simulink model "Tricopter_Controlled_development"  (R2015a)
settings: Solver=ode2  SolverMode=SingleTasking  StartTime=0.0  StopTime=inf  FixedStep=T_sim  RelTol=1e-3
values from neighbouring files (symbols this model uses):
  A_l_max_x = sqrt( (A_z_max)^2  -  g^2  )    [Run3Copter.m]
  A_l_max_y = g*tand(15)    [Run3Copter.m]
  A_x = 0.015    [SetupComplete.m]
  A_y = A_x    (= 0.015)    [SetupComplete.m]
  A_z = 0.16    [SetupComplete.m]
  A_z_max = Max_Thrust*3/m    [Run3Copter.m]
  Alt_0 = input(' Give the initial altitude (m): ')    [Run3Copter.m]
  C_x = 1.2    [SetupComplete.m]
  C_y = C_x    (= 1.2)    [SetupComplete.m]
  C_z = 2.2    [SetupComplete.m]
  CG_0 = [0,0,0.02]'    [SetupComplete.m]
  epsilon = 0.01    [Run3Copter.m]
  eta_23 = deg2rad(-1.3)    [Run3Copter.m]
  g = 9.81    [SetupComplete.m]
  h = 0.08    [SetupComplete.m]
  h_M = 0.064    [SetupComplete.m]
  I_BAC_0 = [ Ix,0,Ixz;0,Iy,0;Ixz,0,Iz]    [SetupComplete.m]
  Initial_Omegas = Omega_hover    [Run3Copter.m]
  Initial_Torques = Torque_hover    [Run3Copter.m]
  Ix = 0.103    [SetupComplete.m]
  Iy = 0.147    [SetupComplete.m]
  Iz = 0.237    [SetupComplete.m]
  l = 0.345    [SetupComplete.m]
  l_arm = 0.264    [SetupComplete.m]
  latitude = 52.071118    [Run3Copter.m]
  longitude = -0.627404    [Run3Copter.m]
  m = 3.51    [SetupComplete.m]
  m_0 = 2.61    [SetupComplete.m]
  m_M = 0.300    (= 0.3)    [SetupComplete.m]
  rho = 1.15    [SetupComplete.m]
  Rotation_sign = [ 1,-1,-1]    [SetupComplete.m]
  T_ctrl = 0.02    [Run3Copter.m]
  T_sim = 0.01    [Run3Copter.m]
  throtle_1 = 0*0.745    (= 0)    [Run3Copter.m]
  throtle_23 = throtle_1/cos(eta_23)    [Run3Copter.m]
  v_i0 = sqrt( 1/3*m*g/(2*rho*pi*R^2)  )    [SetupComplete.m]
undefined symbols (not defined in the file or in its folder): DOWN_0, EAST_0, Newton, NORTH_0, P_0, Q_0, R_0, Raphson, U_0, V_0, W_0
libraries: Adaptive_FaultTolerantControl x30, XXCopter_Control x23, simulink_extras x17, XXCopter x5, simulink x2, qcatlib x1, XXCopter_C x1
(part 2 of 4)

== system Tricopter_Controlled_development/TriCopter FCS development/Build Servos PWM ==
  note: Control input
      | Rango
      | Direccion rot/Dir servos
      | Rango del servo
      |
      | eta_1 (rad) (Pan arm 1)
      | -165,165
      | -1
      | 330: -165,165
      |
      | gamma_1 (rad) (Tilt arm 1)
      | -90,15
      | -1
      | 180:-90,90 ó 330: -165,165
      |
      | eta_2 (rad) (Pan arm 2)
      | -165,165
      | -1
      | 330: -165,165
      |
      | gamma_2 (rad) (Tilt arm 2)
      | -15,90
      | 1
      | 180:-90,90
      |
      | eta_3 (rad) (Pan arm 3)
      | -165,165
      | 1
      | 330:-165,165
      |
      | gamma_3 (rad) (Tilt arm 3)
      | -90,15
      | -1
      | 180:-90,90
  signals servos in : Inport
  Demux : Demux  Outputs=6
  Mux : Mux  Inputs=6
  Signal2PWM1 : XXCopter_Control/Signal2PWM  b=deg2rad(165)  d=-deg2rad(165)  a=2100  c=900
  Signal2PWM2 : XXCopter_Control/Signal2PWM  b=deg2rad(90)  d=-deg2rad(90)  a=2100  c=900
  Signal2PWM3 : XXCopter_Control/Signal2PWM  b=deg2rad(90)  d=-deg2rad(90)  a=2100  c=900
  Signal2PWM4 : XXCopter_Control/Signal2PWM  b=deg2rad(90)  d=-deg2rad(90)  a=2100  c=900
  Signal2PWM5 : XXCopter_Control/Signal2PWM  b=deg2rad(165)  d=-deg2rad(165)  a=2100  c=900
  Signal2PWM6 : XXCopter_Control/Signal2PWM  b=deg2rad(165)  d=-deg2rad(165)  a=2100  c=900
  Unary Minus{,1..3} (4 alike) : UnaryMinus
  PWM_us servos out : Outport
  wires:
  signals servos in/1 -> Demux/1
  Demux/1 -> Unary Minus/1
  Demux/2 -> Unary Minus1/1
  Demux/3 -> Unary Minus2/1
  Demux/6 -> Unary Minus3/1
  Unary Minus3/1 -> Signal2PWM3/1
  Demux/5 -> Signal2PWM6/1
  Demux/4 -> Signal2PWM4/1
  Unary Minus2/1 -> Signal2PWM5/1
  Unary Minus1/1 -> Signal2PWM2/1
  Unary Minus/1 -> Signal2PWM1/1
  Signal2PWM1/1 -> Mux/1
  Signal2PWM2/1 -> Mux/2
  Signal2PWM5/1 -> Mux/3
  Signal2PWM4/1 -> Mux/4
  Signal2PWM6/1 -> Mux/5
  Signal2PWM3/1 -> Mux/6
  Mux/1 -> PWM_us servos out/1

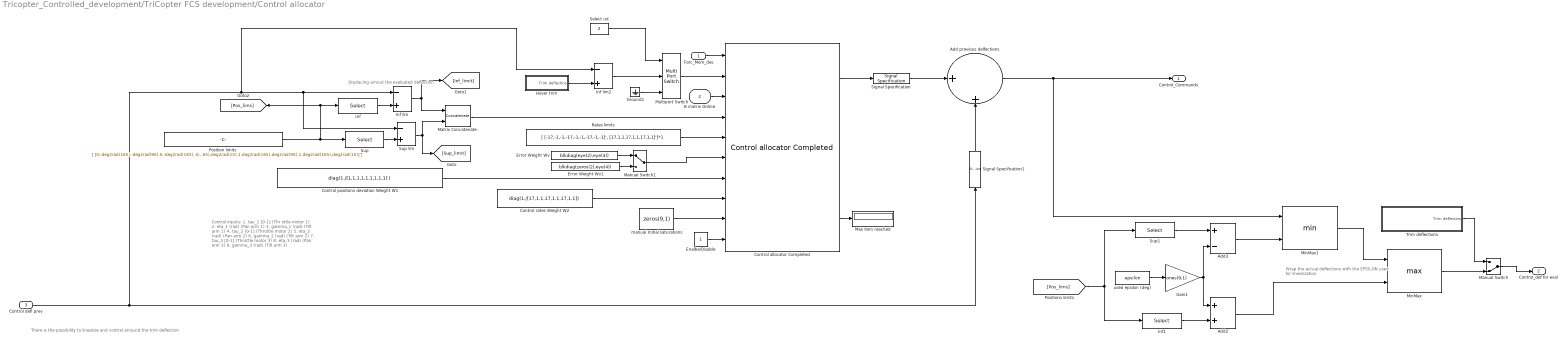
== system Tricopter_Controlled_development/TriCopter FCS development/Control allocator ==
  note: There is the possibility to linearize and control arround the trim deflection
  note: Wrap the actual deflections with the EPSILON
      |  used for linearization
  note: Displacing arroud the evaluated deflection
  note: Control inputs:
      | 1. tau_1 [0-1] (Thr ottle motor 1)
      | 2. eta_1 (rad)  (Pan arm 1)
      | 3. gamma_1 (rad)  (Tilt arm 1)
      |
      | 4. tau_2 [0-1] (Throttle motor 2)
      | 5. eta_2 (rad)  (Pan arm 2)
      | 6. gamma_2 (rad)  (Tilt arm 2)
      |
      | 7. tau_3 [0-1] (Throttle motor 3)
      | 8. eta_3 (rad)  (Pan arm  3)
      | 9. gamma_3 (rad)  (Tilt arm 3)
  Forc_Mom_des : Inport
  B matrix Online : Inport  Port=2
  Control defl prev : Inport  Port=3
  Add previous delfections : Sum  Inputs=|++
  Add2 : Sum
  Add3 : Sum  Inputs=+-
  "Control allocator Completed " : qcatlib/Control allocator Completed   alg=WLS  CA_type=QP  iter_max=100  gamma=1  k_B=6  m_B=9  T=T_ctrl  tol=1e-5
  Control positions deviation Weight W1 : Constant  Value=diag(1./[1,1,1,1,1,1,1,1,1] )
  Control rates Weight W2 : Constant  Value=diag(1./[17,1,1,17,1,1,17,1,1])
  Enalbe/Disable : Constant
  Error Weight Wv : Constant  Value=blkdiag(eye(2),eye(4))
  Error Weight Wv1 : Constant  Value=blkdiag(zeros(2),eye(4))
  Gain1 : Gain  Gain=ones(9,1)
  Ground1 : Ground
  Hover trim : Subsystem  TreatAsAtomicUnit=on
  Inf : Selector  NumberOfDimensions=2  InputPortWidth=3  IndexOptions=Index vector (dialog),Index vector (dialog)  Indices=[1:9],1  OutputSizes=1,1
  Inf lim : Sum  Inputs=-+
  Inf lim2 : Sum  Inputs=-+
  Inf1 : Selector  NumberOfDimensions=2  InputPortWidth=3  IndexOptions=Index vector (dialog),Index vector (dialog)  Indices=[1:9],1  OutputSizes=1,1
  Manual Switch : ManualSwitch  CurrentSetting=0
  Manual Switch1 : ManualSwitch
  Matrix Concatenate : Concatenate  Mode=Multidimensional array  ConcatenateDimension=2
  Max iters reached : Display
  MinMax : MinMax  Function=max  Inputs=2
  MinMax1 : MinMax  Inputs=2
  Multiport Switch : MultiPortSwitch  Inputs=2
  Position limits : Constant  Value=[ [0,-deg2rad(165),-deg2rad(90),0,-deg2rad(165),-deg2rad(15),0,-deg2rad(165),-deg2rad(90)]', [1,deg2rad(165),deg2rad(15),1,deg2rad(165),deg2rad(90),1,deg2rad(165),deg2rad(15)]']
  Rates limits : Constant  Value=[ [-17,-1,-1,-17,-1,-1,-17,-1,-1]', [17,1,1,17,1,1,17,1,1]']*1
  Select ud : Constant  Value=2  SampleTime=-1
  Signal Specification : SignalSpecification  Dimensions=[9,1]
  Signal Specification1 : SignalSpecification  Dimensions=[9,1]
  Sup : Selector  NumberOfDimensions=2  InputPortWidth=3  IndexOptions=Index vector (dialog),Index vector (dialog)  Indices=[1:9],2  OutputSizes=1,1
  Sup lim : Sum  Inputs=-+
  Sup1 : Selector  NumberOfDimensions=2  InputPortWidth=3  IndexOptions=Index vector (dialog),Index vector (dialog)  Indices=[1:9],2  OutputSizes=1,1
  Trim deflections : Subsystem  TreatAsAtomicUnit=on
  manual Initial saturations : Constant  Value=zeros(9,1)
  used epsilon (deg) : Constant  Value=epsilon
  Control_Commands : Outport
  Control_def for eval : Outport  Port=2
  wires:
  Manual Switch/1 -> Control_def for eval/1
  MinMax1/1 -> MinMax/1
  Add3/1 -> MinMax1/2
  used epsilon (deg)/1 -> Gain1/1
  Inf1/1 -> Add2/2
  Gain1/1 -> Add3/2, Add2/1
  Sup1/1 -> Add3/1
  Add2/1 -> MinMax/2
  Control positions deviation Weight W1/1 -> "Control allocator Completed "/7
  "Control allocator Completed "/1 -> Signal Specification/1
  Enalbe/Disable/1 -> "Control allocator Completed "/10
  manual Initial saturations/1 -> "Control allocator Completed "/9
  "Control allocator Completed "/3 -> Max iters reached/1
  Sup lim/1 -> [Sup_limit], Matrix Concatenate/2
  Inf lim/1 -> [Inf_limit], Matrix Concatenate/1
  Inf/1 -> Inf lim/2
  Sup/1 -> Sup lim/2
  Control rates Weight W2/1 -> "Control allocator Completed "/8
  Manual Switch1/1 -> "Control allocator Completed "/6
  Rates limits/1 -> "Control allocator Completed "/5
  Add previous delfections/1 -> Control_Commands/1, MinMax1/1
  B matrix Online/1 -> "Control allocator Completed "/3
  Signal Specification/1 -> Add previous delfections/1
  Signal Specification1/1 -> Add previous delfections/2
  [Pos_lims] -> Sup1/1, Inf1/1
  Forc_Mom_des/1 -> "Control allocator Completed "/1
  Trim deflections/1(Trim deflectins) -> Manual Switch/1
  MinMax/1 -> Manual Switch/2
  Matrix Concatenate/1 -> "Control allocator Completed "/4
  Multiport Switch/1 -> "Control allocator Completed "/2
  Error Weight Wv/1 -> Manual Switch1/1
  Error Weight Wv1/1 -> Manual Switch1/2
  Hover trim/1(Trim deflectins) -> Inf lim2/2
  Control defl prev/1 -> Signal Specification1/1, Inf lim2/1, Inf lim/1, Sup lim/1
  Inf lim2/1 -> Multiport Switch/2
  Select ud/1 -> Multiport Switch/1
  Position limits/1 -> [Pos_lims], Inf/1, Sup/1
  Ground1/1 -> Multiport Switch/3

== system Tricopter_Controlled_development/TriCopter FCS development/Inner Controller ==
  note: 1) Only subsystems can be added as variant choices at this level
      | 2) Blocks cannot be connected at this level as connectivity is
      | automatically determined at simulation, based on the active variant
  Accels ref (m/s^2) : Inport
  Phi_ref (rad) : Inport  Port=2
  Theta_ref (rad) : Inport  Port=3
  Yaw_ref (rad) : Inport  Port=4
  All meas : Inport  Port=5
  P Controller : Subsystem  VariantControl=P
  PI Controller : Subsystem  VariantControl=PI
  PI Controller Quaternions : Subsystem  VariantControl=PI_quat
  Accs_Ang_acc des : Outport

== system Tricopter_Controlled_development/TriCopter FCS development/NDI ==
  note: Rejection for the
      | angular accelerations
  note: Pseudo control inputs:
      | 1. Desired angular accelerations (rad/s^2)
      | 2. Desired accelerations (m/s^2) in body axes
  pseudo_control (m/s^2;rad/s^2) : Inport
  Control_defl for eval : Inport  Port=2
  m : Inport  Port=3
  All_meas : Inport  Port=4
  3Copter_4_NDI&CA : Subsystem  AncestorBlock=XXCopter_Control/3Copter_4_NDI&CA  TreatAsAtomicUnit=on
  Bus Selector : BusSelector  OutputSignals=Meas.omega_b meas (rad/s),Meas.q_meas,Meas.V_b_meas,Meas.Alt meas (m)
  Demux : Demux  Outputs=[3,3]
  Derivative1 : Derivative  CoefficientInTFapproximation=500
  Ground : Ground
  Ground1 : Ground
  Inversion : Sum  Inputs=|+-
  Mux : Mux  Inputs=[3,3]
  Mux2 : Mux  Inputs=[3,3]
  Rot eqs_ Get moments : XXCopter_Control/Rot eqs_ Get moments
  Transl Eqs_ Get forces : XXCopter_Control/Transl Eqs_ Get forces
  "angles " : Selector  IndexMode=Zero-based  InputPortWidth=9  Indices=[1,2,4,5,7,8]
  epsilon (rad or unitary) : Constant  Value=epsilon
  m1 : InportShadow  Port=3
  Virtual Control Commands : Outport
  B online : Outport  Port=2
  Control_defl eval (rad) : Outport  Port=3
  wires:
  3Copter_4_NDI&CA/3(CA_grad) -> B online/1
  Mux/1 -> Inversion/1
  Mux2/1 -> Inversion/2  "f_x(x)"
  All_meas/1 -> Bus Selector/1
  pseudo_control (m/s^2;rad/s^2)/1 -> Demux/1
  Demux/2 -> Rot eqs_ Get moments/2, Transl Eqs_ Get forces/4
  Demux/1 -> Transl Eqs_ Get forces/1
  Bus Selector/1 -> Transl Eqs_ Get forces/3, Rot eqs_ Get moments/1, 3Copter_4_NDI&CA/6(omega_b)  "<omega_b meas (rad/s)>"
  Bus Selector/3 -> Transl Eqs_ Get forces/2, 3Copter_4_NDI&CA/4(Vb)  "<V_b_meas>"
  3Copter_4_NDI&CA/4(I_BAC) -> Rot eqs_ Get moments/3
  3Copter_4_NDI&CA/5("CG ") -> Transl Eqs_ Get forces/6
  Control_defl for eval/1 -> 3Copter_4_NDI&CA/2(Control Inputs (rad)), Control_defl eval (rad)/1, "angles "/1
  Bus Selector/4 -> 3Copter_4_NDI&CA/3(h)  "<Alt meas (m)>"
  Bus Selector/2 -> 3Copter_4_NDI&CA/5(q)  "<q_meas>"
  m/1 -> 3Copter_4_NDI&CA/11(" m")
  m1/1 -> Transl Eqs_ Get forces/5
  epsilon (rad or unitary)/1 -> 3Copter_4_NDI&CA/1("epsilon (rad or unitary) ")
  Transl Eqs_ Get forces/1 -> Mux/1
  Rot eqs_ Get moments/1 -> Mux/2
  3Copter_4_NDI&CA/1(Forces) -> Mux2/1
  3Copter_4_NDI&CA/2(Moments) -> Mux2/2
  Inversion/1 -> Virtual Control Commands/1
  Ground/1 -> 3Copter_4_NDI&CA/7(Omegas_dot_actual)
  "angles "/1 -> Derivative1/1, 3Copter_4_NDI&CA/8(angles_actual)
  Derivative1/1 -> 3Copter_4_NDI&CA/9(angles_dot_actual)
  Ground1/1 -> 3Copter_4_NDI&CA/10(angles_dot_dot_actual)

== system Tricopter_Controlled_development/TriCopter FCS development/Outer Controller ==
  note: 1) Only subsystems can be added as variant choices at this level
      | 2) Blocks cannot be connected at this level as connectivity is
      | automatically determined at simulation, based on the active variant
  Position ref (m) : Inport
  Attitude ref (rad) : Inport  Port=2
  Yaw_ref (rad) : Inport  Port=3
  All meas : Inport  Port=4
  Overactuated P Controller : Subsystem  VariantControl=Overactuated P Controller
  Underactuated P Controller : Subsystem  VariantControl=Underactuated P Controller
  Accels des : Outport
  Euler des : Outport  Port=2

== system Tricopter_Controlled_development/TriCopter FCS development/keep -90//90 ==
  in (rad) : Inport
  Constant : Constant  Value=180
  Constant2 : Constant  Value=360
  Gain : Gain  Gain=360
  Math Function2 : Math  Operator=rem  SaturateOnIntegerOverflow=on
  Product : Product  Inputs=*/  RndMeth=Zero
  Rounding Function : Rounding  Operator=fix
  Sum2 : Sum  Inputs=|-+
  deg2rad1 : Gain  Gain=pi/180  SaturateOnIntegerOverflow=on  OutDataTypeStr=Inherit: Same as input  ParamDataTypeStr=Inherit: Same as input
  rad2deg : Gain  Gain=180/pi  SaturateOnIntegerOverflow=on  OutDataTypeStr=Inherit: Same as input  ParamDataTypeStr=Inherit: Same as input
  out (rad) : Outport
  wires:
  deg2rad1/1 -> out (rad)/1
  Sum2/1 -> deg2rad1/1
  Math Function2/1 -> Sum2/2, Product/1
  Constant2/1 -> Math Function2/2
  rad2deg/1 -> Math Function2/1
  Gain/1 -> Sum2/1
  Rounding Function/1 -> Gain/1
  Product/1 -> Rounding Function/1
  Constant/1 -> Product/2
  in (rad)/1 -> rad2deg/1

== system Tricopter_Controlled_development/3 Copter Complete/6dof Eqs of motion/DCM1 ==
  Euler : Inport  PortDimensions=3
  Fcn11 : Fcn  Expr=u(5)*u(4)
  Fcn12 : Fcn  Expr=u(5)*u(1)
  Fcn13 : Fcn  Expr=-u(2)
  Fcn21 : Fcn  Expr=u(3)*u(2)*u(4) - u(6)*u(1)
  Fcn22 : Fcn  Expr=u(3)*u(2)*u(1) + u(6)*u(4)
  Fcn23 : Fcn  Expr=u(3)*u(5)
  Fcn31 : Fcn  Expr=u(6)*u(2)*u(4) + u(3)*u(1)
  Fcn32 : Fcn  Expr=u(6)*u(2)*u(1) - u(3)*u(4)
  Fcn33 : Fcn  Expr=u(6)*u(5)
  Mux : Mux  Inputs=2
  Mux1 : Mux  Inputs=9
  Reshape : Reshape  OutputDimensionality=Customize  OutputDimensions=[3,3]
  sincos : Trigonometry  Operator=sincos
  DCM : Outport  PortDimensions=[3,3]
  wires:
  Fcn33/1 -> Mux1/9
  Fcn32/1 -> Mux1/8
  Fcn23/1 -> Mux1/6
  Fcn22/1 -> Mux1/5
  Fcn31/1 -> Mux1/7
  Fcn21/1 -> Mux1/4
  Fcn13/1 -> Mux1/3
  Fcn12/1 -> Mux1/2
  Fcn11/1 -> Mux1/1
  Mux/1 -> Fcn22/1, Fcn23/1, Fcn31/1, Fcn33/1, Fcn32/1, Fcn21/1, Fcn13/1, Fcn12/1, Fcn11/1
  sincos/2 -> Mux/2
  sincos/1 -> Mux/1
  Reshape/1 -> DCM/1
  Euler/1 -> sincos/1
  Mux1/1 -> Reshape/1

== system Tricopter_Controlled_development/3 Copter Complete/6dof Eqs of motion/q_dot ==
  note: Both of these methods to compute q_dot are very similar
  omega_b : Inport
  q : Inport  Port=2
  Quaternion_dot : MATLAB Function  TreatAsAtomicUnit=on  VariantControl=Variant
  q_dot : Outport
  wires:
  omega_b/1 -> Quaternion_dot/1(omega_b)  "omega_b"
  q/1 -> Quaternion_dot/2(q)  "q"
  Quaternion_dot/1(q_dot) -> q_dot/1

== system Tricopter_Controlled_development/FlightGear visualization/Flat Earth to LLA/ne to lat//long ==
  Xe : Inport
  Demux : Demux  Outputs=2
  "Latitude Between +/- 90 " : Subsystem  TreatAsAtomicUnit=on
  "LongLat_offset " : Subsystem  TreatAsAtomicUnit=on
  "Longitude Between +/-180 " : Subsystem  TreatAsAtomicUnit=on
  Sel1 : Selector  InputPortWidth=3  Indices=[1,2]
  Sum2 : Sum  Inputs=++|
  initial_latg : Constant  Value=latitude
  initial_pos : Constant  Value=[latitude,longitude]
  rad2deg : Gain  Gain=180/pi  SaturateOnIntegerOverflow=on  OutDataTypeStr=Inherit: Same as input  ParamDataTypeStr=Inherit: Same as input
  lat_deg : Outport
  long_deg : Outport  Port=2
  wires:
  Xe/1 -> Sel1/1
  Sum2/1 -> "Latitude Between +/- 90 "/1(mu l)
  "LongLat_offset "/1(DeltaLL_rad) -> rad2deg/1
  Sel1/1 -> "LongLat_offset "/1(XY)
  rad2deg/1 -> Sum2/2
  initial_pos/1 -> Sum2/1
  initial_latg/1 -> "LongLat_offset "/2(mu)
  "Latitude Between +/- 90 "/1("mu l ") -> "Longitude Between +/-180 "/1(mu l)
  "Longitude Between +/-180 "/1("mu l ") -> Demux/1
  Demux/1 -> lat_deg/1
  Demux/2 -> long_deg/1

== system Tricopter_Controlled_development/Sensors and filtering. No noise/Sensors and filtering. No noise/keep -pi//pi1 ==
  in (rad) : Inport
  Constant : Constant  Value=180
  Constant2 : Constant  Value=360
  Gain : Gain  Gain=360
  Math Function2 : Math  Operator=rem  SaturateOnIntegerOverflow=on
  Product : Product  Inputs=*/  RndMeth=Zero
  Rounding Function : Rounding  Operator=fix
  Sum2 : Sum  Inputs=|-+
  deg2rad1 : Gain  Gain=pi/180  SaturateOnIntegerOverflow=on  OutDataTypeStr=Inherit: Same as input  ParamDataTypeStr=Inherit: Same as input
  rad2deg : Gain  Gain=180/pi  SaturateOnIntegerOverflow=on  OutDataTypeStr=Inherit: Same as input  ParamDataTypeStr=Inherit: Same as input
  out (rad) : Outport
  wires:
  deg2rad1/1 -> out (rad)/1
  Sum2/1 -> deg2rad1/1
  Math Function2/1 -> Sum2/2, Product/1
  Constant2/1 -> Math Function2/2
  rad2deg/1 -> Math Function2/1
  Gain/1 -> Sum2/1
  Rounding Function/1 -> Gain/1
  Product/1 -> Rounding Function/1
  Constant/1 -> Product/2
  in (rad)/1 -> rad2deg/1

== system Tricopter_Controlled_development/Sensors and filtering. No noise/Sensors and filtering. Noise/keep -pi//pi1 ==
  in (rad) : Inport
  Constant : Constant  Value=180
  Constant2 : Constant  Value=360
  Gain : Gain  Gain=360
  Math Function2 : Math  Operator=rem  SaturateOnIntegerOverflow=on
  Product : Product  Inputs=*/  RndMeth=Zero
  Rounding Function : Rounding  Operator=fix
  Sum2 : Sum  Inputs=|-+
  deg2rad1 : Gain  Gain=pi/180  SaturateOnIntegerOverflow=on  OutDataTypeStr=Inherit: Same as input  ParamDataTypeStr=Inherit: Same as input
  rad2deg : Gain  Gain=180/pi  SaturateOnIntegerOverflow=on  OutDataTypeStr=Inherit: Same as input  ParamDataTypeStr=Inherit: Same as input
  out (rad) : Outport
  wires:
  deg2rad1/1 -> out (rad)/1
  Sum2/1 -> deg2rad1/1
  Math Function2/1 -> Sum2/2, Product/1
  Constant2/1 -> Math Function2/2
  rad2deg/1 -> Math Function2/1
  Gain/1 -> Sum2/1
  Rounding Function/1 -> Gain/1
  Product/1 -> Rounding Function/1
  Constant/1 -> Product/2
  in (rad)/1 -> rad2deg/1

== system Tricopter_Controlled_development/TriCopter FCS development/Control allocator/Hover trim ==
  Ground1 : Ground
  Trim state : Bias  Bias=[throtle_1,0,0,throtle_23,eta_23,0,throtle_23,-eta_23,0]'
  Trim deflectins : Outport
  wires:
  Trim state/1 -> Trim deflectins/1
  Ground1/1 -> Trim state/1

== system Tricopter_Controlled_development/TriCopter FCS development/Control allocator/Trim deflections ==
  Contro Inputs1 : Constant  Value=throtle_1
  Contro Inputs2 : Constant  Value=throtle_23
  Contro Inputs3 : Constant  Value=eta_23
  Gain : Gain  Gain=-1
  Ground : Ground
  Mux : Mux  Inputs=9
  Trim deflectins : Outport
  wires:
  Contro Inputs1/1 -> Mux/1
  Contro Inputs2/1 -> Mux/7, Mux/4
  Ground/1 -> Mux/2, Mux/6, Mux/9, Mux/3
  Contro Inputs3/1 -> Gain/1, Mux/5
  Gain/1 -> Mux/8
  Mux/1 -> Trim deflectins/1

== system Tricopter_Controlled_development/TriCopter FCS development/Inner Controller/P Controller ==
  note: These limits are wrong?
  note: Limits here for the maximum asymetrical thortle deflection
  Accels ref (m/s^2) : Inport
  Phi_ref (rad) : Inport  Port=2
  Theta_ref (rad) : Inport  Port=3
  Yaw_ref (rad) : Inport  Port=4
  All meas : Inport  Port=5
  Attitude Controller : Subsystem
  Body Rates Controller : Subsystem
  Bus Selector : BusSelector  OutputSignals=Meas.Euler meas (rad)
  Demux : Demux  Outputs=3
  MATLAB Function : MATLAB Function  TreatAsAtomicUnit=on
  Mux : Mux  Inputs=2
  Saturation : Saturate  UpperLimit=[0.4,0.4,0.1]'  LowerLimit=-[0.4,0.4,0.1]'
  Saturation1 : Saturate  UpperLimit=deg2rad(45)/5*[2,2,1]'  LowerLimit=-deg2rad(45)/5*[2,2,1]'
  Accs_Ang_acc des : Outport
  wires:
  Accels ref (m/s^2)/1 -> Mux/1
  Body Rates Controller/1(Angular acc des (rad/s^2)) -> Saturation/1
  MATLAB Function/1(Omega) -> Demux/1
  Mux/1 -> Accs_Ang_acc des/1
  Attitude Controller/1(Euler_dot des (rad/s)) -> Saturation1/1
  All meas/1 -> Attitude Controller/4(All_meas), Body Rates Controller/4(All_meas), Bus Selector/1
  Phi_ref (rad)/1 -> Attitude Controller/1(phi_ref)
  Yaw_ref (rad)/1 -> Attitude Controller/3(psi_ref)
  Theta_ref (rad)/1 -> Attitude Controller/2(theta_ref)
  Bus Selector/1 -> MATLAB Function/2(euler_ang)  "<Euler meas (rad)>"
  Demux/1 -> Body Rates Controller/1(p_ref)
  Demux/2 -> Body Rates Controller/2(q_ref)
  Demux/3 -> Body Rates Controller/3(r_ref)
  Saturation/1 -> Mux/2
  Saturation1/1 -> MATLAB Function/1(ang_dot)

== system Tricopter_Controlled_development/TriCopter FCS development/Inner Controller/PI Controller ==
  note: Limits here for the maximum asymetrical thortle deflection
  Accels ref (m/s^2) : Inport
  Phi_ref (rad) : Inport  Port=2
  Theta_ref (rad) : Inport  Port=3
  Yaw_ref (rad) : Inport  Port=4
  All meas : Inport  Port=5
  Attitude Controller : Subsystem
  Body Rates Controller : Subsystem
  Bus Selector : BusSelector  OutputSignals=Meas.Euler meas (rad)
  Demux : Demux  Outputs=3
  Limits in Ang accel : Subsystem  TreatAsAtomicUnit=on
  MATLAB Function : MATLAB Function  TreatAsAtomicUnit=on
  Mux : Mux  Inputs=2
  Saturation1 : Saturate  UpperLimit=deg2rad(20)*[1,1,0.5]'  LowerLimit=-deg2rad(20)*[1,1,0.5]'
  keep -pi/pi1 : Subsystem
  keep -pi/pi2 : Subsystem
  keep -pi/pi3 : Subsystem
  Accs_Ang_acc des : Outport
  wires:
  Limits in Ang accel/1(ang Ace des) -> Mux/2
  Demux/3 -> Body Rates Controller/3(r_ref)
  Demux/2 -> Body Rates Controller/2(q_ref)
  Demux/1 -> Body Rates Controller/1(p_ref)
  Bus Selector/1 -> Limits in Ang accel/2(Euler meas), MATLAB Function/2(euler_ang)  "<Euler meas (rad)>"
  Theta_ref (rad)/1 -> keep -pi/pi2/1(in (rad))
  Yaw_ref (rad)/1 -> keep -pi/pi3/1(in (rad))
  Phi_ref (rad)/1 -> keep -pi/pi1/1(in (rad))
  All meas/1 -> Body Rates Controller/4(All_meas), Bus Selector/1, Attitude Controller/4(All_meas)
  Mux/1 -> Accs_Ang_acc des/1
  MATLAB Function/1(Omega) -> Demux/1
  Accels ref (m/s^2)/1 -> Mux/1
  Body Rates Controller/1(Angular acc des (rad/s^2)) -> Limits in Ang accel/1(Ang Ace des)
  keep -pi/pi1/1(out (rad)) -> Attitude Controller/1(phi_ref)
  keep -pi/pi2/1(out (rad)) -> Attitude Controller/2(theta_ref)
  keep -pi/pi3/1(out (rad)) -> Attitude Controller/3(psi_ref)
  Attitude Controller/1(Euler_dot des (rad/s)) -> Saturation1/1
  Saturation1/1 -> MATLAB Function/1(ang_dot)

== system Tricopter_Controlled_development/TriCopter FCS development/Inner Controller/PI Controller Quaternions ==
  note: Limits here
  note: Limits here for the maximum asymetrical thortle deflection
  Accels ref (m/s^2) : Inport
  Phi_ref (rad) : Inport  Port=2
  Theta_ref (rad) : Inport  Port=3
  Yaw_ref (rad) : Inport  Port=4
  All meas : Inport  Port=5
  Add : Sum
  Add1 : Sum  Inputs=+-
  Add2 : Sum  Inputs=+-
  Attitude Controller : Subsystem
  Body Rates Controller : Subsystem
  Bus Selector : BusSelector  OutputSignals=Meas.Euler meas (rad)
  Bus Selector1 : BusSelector  OutputSignals=Meas.q_meas
  Demux : Demux  Outputs=3
  Get Quaternion from des euler : MATLAB Function  TreatAsAtomicUnit=on
  Limits in Ang accel : Subsystem  TreatAsAtomicUnit=on
  MATLAB Function : MATLAB Function  TreatAsAtomicUnit=on
  Mux : Mux  Inputs=2
  Quaternion_dot : MATLAB Function  TreatAsAtomicUnit=on  VariantControl=Variant
  Saturation1 : Saturate  UpperLimit=deg2rad(50)*[1,10,0.5]'  LowerLimit=-deg2rad(50)*[1,10,0.5]'
  Scope : Scope  NumInputPorts=2
      settings: YMin=-0.5~-0.5  YMax=2.25~2.25  SaveName=ScopeData7
  T : Gain  Gain=T_ctrl
  Accs_Ang_acc des : Outport
  wires:
  Accels ref (m/s^2)/1 -> Mux/1
  Mux/1 -> Accs_Ang_acc des/1
  All meas/1 -> Bus Selector/1, Attitude Controller/5(All_meas), Body Rates Controller/4(All_meas), Bus Selector1/1
  Bus Selector/1 -> Limits in Ang accel/2(Euler meas), MATLAB Function/2(Euler)  "<Euler meas (rad)>"
  Demux/1 -> Body Rates Controller/1(p_ref)
  Demux/2 -> Body Rates Controller/2(q_ref)
  Demux/3 -> Body Rates Controller/3(r_ref)
  Phi_ref (rad)/1 -> Attitude Controller/2(Phi_ref (rad)), Get Quaternion from des euler/1(phi)
  Theta_ref (rad)/1 -> Get Quaternion from des euler/2(theta)
  Yaw_ref (rad)/1 -> Attitude Controller/4(Yaw_ref (rad)), Get Quaternion from des euler/3(psi)
  Bus Selector1/1 -> Quaternion_dot/2(q)  "<q_meas>"
  Get Quaternion from des euler/1(q) -> Attitude Controller/3(q_ref)
  Attitude Controller/1(quat_dot des (rad/s)) -> Quaternion_dot/1(q_dot)
  Saturation1/1 -> Add1/1, Demux/1
  Limits in Ang accel/1(ang Ace des) -> Scope/2, Add2/1, Mux/2
  Quaternion_dot/1(omega_b) -> Add1/2, Saturation1/1
  Body Rates Controller/1(Angular acc des (rad/s^2)) -> Limits in Ang accel/1(Ang Ace des), Add2/2, Scope/1
  Add/1 -> MATLAB Function/1(omega_b)
  Add2/1 -> T/1
  Add1/1 -> Add/2
  T/1 -> Add/1
  MATLAB Function/1(Euler_dot) -> Attitude Controller/1(AWU)

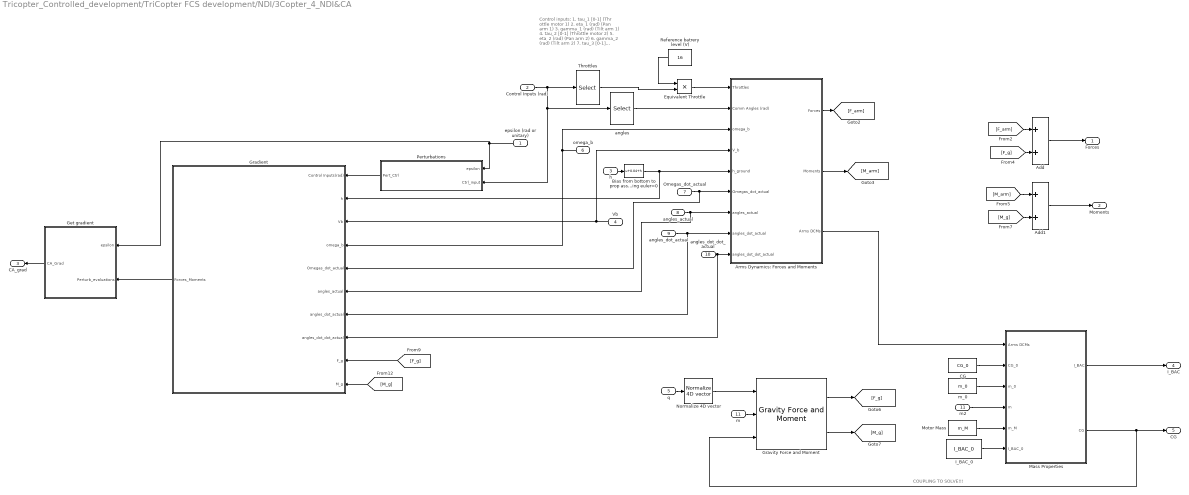
== system Tricopter_Controlled_development/TriCopter FCS development/NDI/3Copter_4_NDI&CA ==
  note: Control inputs:
      | 1. tau_1 [0-1] (Thr ottle motor 1)
      | 2. eta_1 (rad)  (Pan arm 1)
      | 3. gamma_1 (rad)  (Tilt arm 1)
      |
      | 4. tau_2 [0-1] (Throttle motor 2)
      | 5. eta_2 (rad)  (Pan arm 2)
      | 6. gamma_2 (rad)  (Tilt arm 2)
      |
      | 7. tau_3 [0-1] (Throttle motor 3)
      | 8. eta_3 (rad)  (Pan arm  3)
      | 9. gamma_3 (rad)  (Tilt arm 3)
  note: COUPLING TO SOLVE!!!
  "epsilon (rad or unitary) " : Inport
  Control Inputs (rad) : Inport  Port=2
  h : Inport  Port=3
  Vb : Inport  Port=4
  q : Inport  Port=5
  omega_b : Inport  Port=6
  Omegas_dot_actual : Inport  Port=7
  angles_actual : Inport  Port=8
  angles_dot_actual : Inport  Port=9
  angles_dot_dot_actual : Inport  Port=10
  " m" : Inport  Port=11
  Add : Sum
  Add1 : Sum
  Arms Dynamics: Forces and Moments : Subsystem  TreatAsAtomicUnit=on
  Bias from bottom to prop assuming euler=0 : Bias  Bias=0.04+h
  CG : Constant  Value=CG_0
  Equivalent Throttle : Product  Inputs=**
  Get gradient : MATLAB Function  TreatAsAtomicUnit=on
  Gradient : Subsystem  TreatAsAtomicUnit=on
  Gravity Force and Moment : XXCopter_Control/Gravity Force and Moment
  I_BAC_0 : Constant  Value=I_BAC_0
  Mass Properties : Subsystem  TreatAsAtomicUnit=on
  Motor Mass : Constant  Value=m_M
  Normalize 4D vector : XXCopter/Normalize 4D vector
  Perturbations : MATLAB Function  TreatAsAtomicUnit=on
  Reference batrery level (V) : Constant  Value=16
  Throttles : Selector  IndexMode=Zero-based  InputPortWidth=9  Indices=[0,3,6]
  "angles " : Selector  IndexMode=Zero-based  InputPortWidth=9  Indices=[1,2,4,5,7,8]
  m2 : InportShadow  Port=11
  m_0 : Constant  Value=m_0
  Forces : Outport
  Moments : Outport  Port=2
  CA_grad : Outport  Port=3
  I_BAC : Outport  Port=4
  "CG " : Outport  Port=5
  wires:
  Get gradient/1(CA_Grad) -> CA_grad/1
  "epsilon (rad or unitary) "/1 -> Perturbations/1(epsilon), Get gradient/1(epsilon)
  Perturbations/1(Pert_Ctrl) -> Gradient/1("Control Inputs(rad) ")
  Gradient/1(Forces_Moments) -> Get gradient/2(Perturb_evaluations)
  Mass Properties/1(I_BAC) -> I_BAC/1
  [F_g] -> Gradient/9(F_g)
  [M_g] -> Gradient/10(M_g)
  Normalize 4D vector/1 -> Gravity Force and Moment/1
  angles_dot_actual/1 -> Arms Dynamics: Forces and Moments/8(angles_dot_actual), Gradient/7(angles_dot_actual)
  Omegas_dot_actual/1 -> Gradient/5(Omegas_dot_actual), Arms Dynamics: Forces and Moments/6(Omegas_dot_actual)
  q/1 -> Normalize 4D vector/1
  Add1/1 -> Moments/1
  Reference batrery level (V)/1 -> Equivalent Throttle/1
  Equivalent Throttle/1 -> Arms Dynamics: Forces and Moments/1(Throttles)
  Mass Properties/2(CG) -> Gravity Force and Moment/3, "CG "/1
  Add/1 -> Forces/1
  m2/1 -> Mass Properties/4(m)
  m_0/1 -> Mass Properties/3(m_0)
  I_BAC_0/1 -> Mass Properties/6(I_BAC_0)
  Motor Mass/1 -> Mass Properties/5(m_M)
  CG/1 -> Mass Properties/2(CG_0)
  Arms Dynamics: Forces and Moments/3(Arms DCMs) -> Mass Properties/1(Arms DCMs)
  Control Inputs (rad)/1 -> Throttles/1, Perturbations/2(Ctrl_input), "angles "/1
  Throttles/1 -> Equivalent Throttle/2
  [M_g] -> Add1/2
  [M_arm] -> Add1/1
  [F_g] -> Add/2
  [F_arm] -> Add/1
  Gravity Force and Moment/2 -> [M_g]
  Gravity Force and Moment/1 -> [F_g]
  Arms Dynamics: Forces and Moments/2(Moments) -> [M_arm]
  Arms Dynamics: Forces and Moments/1(Forces) -> [F_arm]
  " m"/1 -> Gravity Force and Moment/2
  omega_b/1 -> Gradient/4(omega_b), Arms Dynamics: Forces and Moments/3(omega_b)
  Vb/1 -> Arms Dynamics: Forces and Moments/4(V_b), Gradient/3(Vb)
  angles_actual/1 -> Gradient/6(angles_actual), Arms Dynamics: Forces and Moments/7(angles_actual)
  "angles "/1 -> Arms Dynamics: Forces and Moments/2(Comm Angles (rad))
  angles_dot_dot_actual/1 -> Gradient/8(angles_dot_dot_actual), Arms Dynamics: Forces and Moments/9(angles_dot_dot_actual)
  h/1 -> Bias from bottom to prop assuming euler=0/1
  Bias from bottom to prop assuming euler=0/1 -> Arms Dynamics: Forces and Moments/5(h_ground), Gradient/2(h)

== system Tricopter_Controlled_development/TriCopter FCS development/Outer Controller/Overactuated P Controller ==
  Position ref (m) : Inport
  Attitude ref (rad) : Inport  Port=2
  Yaw_ref (rad) : Inport  Port=3
  All meas : Inport  Port=4
  AWU : Product  Multiplication=Matrix(*)
  Add : Sum
  Add1 : Sum  Inputs=+-
  Add2 : Sum  Inputs=+-
  Bus Selector : BusSelector  OutputSignals=Meas.V_e_meas
  Bus Selector1 : BusSelector  OutputSignals=Meas.Euler meas (rad),Params.DCM
  Demux1 : Demux  Outputs=3
  Demux2 : Demux  Outputs=3
  MATLAB Function : MATLAB Function  TreatAsAtomicUnit=on
  Matrix Multiply{1..4} (4 alike) : Product  Multiplication=Matrix(*)
  Permute Dimensions : PermuteDimensions
  Permute Dimensions1 : PermuteDimensions
  Permute Dimensions2 : PermuteDimensions
  Position Controller : Subsystem
  Saturation : Saturate  UpperLimit=[A_l_max_x,A_l_max_y,g]  LowerLimit=-[A_l_max_x,A_l_max_y,A_z_max-g]
  Saturation1 : Saturate  UpperLimit=[10,10,v_i0]  LowerLimit=-[10,10,2*v_i0]
  Selector1 : Selector  InputPortWidth=3  Indices=3
  T : Gain  Gain=T_ctrl
  Terminator : Terminator
  Velocity Controller : Subsystem
  Accels des : Outport
  Euler des : Outport  Port=2
  wires:
  Demux2/3 -> Velocity Controller/3(Vyaw_z_ref)
  Demux2/1 -> Velocity Controller/1(Vyaw_x_ref)
  Demux2/2 -> Velocity Controller/2(Vyaw_y_ref)
  Attitude ref (rad)/1 -> Euler des/1
  All meas/1 -> Position Controller/5(All_meas), Bus Selector1/1, Bus Selector/1
  Position ref (m)/1 -> Demux1/1
  Demux1/3 -> Position Controller/4(X_e_z_ref)
  Demux1/2 -> Position Controller/3(X_e_y_ref)
  Demux1/1 -> Position Controller/2(X_e_x_ref)
  Bus Selector1/2 -> Permute Dimensions/1  "<DCM>"
  Matrix Multiply1/1 -> Accels des/1
  Permute Dimensions/1 -> Matrix Multiply1/1
  Yaw_ref (rad)/1 -> Terminator/1
  Selector1/1 -> MATLAB Function/1(yaw)
  Bus Selector1/1 -> Selector1/1  "<Euler meas (rad)>"
  Position Controller/1(Ve des (m/s)) -> Matrix Multiply2/2
  Saturation1/1 -> Add1/1, Demux2/1
  Saturation/1 -> Add2/1, Matrix Multiply3/2
  MATLAB Function/1(T_yaw) -> Permute Dimensions1/1, Permute Dimensions2/1, Matrix Multiply2/1, Matrix Multiply4/1
  Matrix Multiply2/1 -> Add1/2, Saturation1/1
  Matrix Multiply3/1 -> Matrix Multiply1/2  "in F_e"
  Permute Dimensions1/1 -> Matrix Multiply3/1
  Matrix Multiply4/1 -> Velocity Controller/4(V_yaw_meas)
  Bus Selector/1 -> Matrix Multiply4/2  "<V_e_meas>"
  Velocity Controller/1(Acc_yaw des (m/s)) -> Add2/2, Saturation/1
  Permute Dimensions2/1 -> AWU/1
  Add/1 -> AWU/2
  Add2/1 -> T/1
  Add1/1 -> Add/2
  AWU/1 -> Position Controller/1(AWU)
  T/1 -> Add/1

== system Tricopter_Controlled_development/TriCopter FCS development/Outer Controller/Underactuated P Controller ==
  note: This can be considered as a Guidance module!!!!!!!!!
  note: Limiter here i Acceleration magnitude!!!!!!!
  Position ref (m) : Inport
  Attitude ref (rad) : Inport  Port=2
  Yaw_ref (rad) : Inport  Port=3
  All meas : Inport  Port=4
  3D vec norm : XXCopter_C/3D vec norm
  A_x : Selector  InputPortWidth=3
  A_y : Selector  InputPortWidth=3  Indices=2
  Bus Selector1 : BusSelector  OutputSignals=Meas.Euler meas (rad)
  Demux1 : Demux  Outputs=3
  Demux2 : Demux  Outputs=3
  Divide : Product  Inputs=*/
  Divide1 : Product  Inputs=/*
  Gain : Gain  Gain=-1
  Mux1 : Mux  Inputs=2
  Mux2 : Mux  Inputs=3
  Position Controller : Subsystem
  Selector : Selector  InputPortWidth=3  Indices=3
  Terminator : Terminator
  Trigonometric Function : Trigonometry  Operator=atan
  Trigonometric Function1 : Trigonometry  Operator=atan
  Velocity Controller : Subsystem
  Yaw rotate : MATLAB Function  TreatAsAtomicUnit=on
  Zero in accels : Constant  Value=[0,0]
  g : Constant  Value=g
  Accels des : Outport
  Euler des : Outport  Port=2
  wires:
  Zero in accels/1 -> Mux1/1
  Demux1/1 -> Position Controller/1(X_e_x_ref)
  Demux1/2 -> Position Controller/2(X_e_y_ref)
  Demux1/3 -> Position Controller/3(X_e_z_ref)
  Position ref (m)/1 -> Demux1/1
  Attitude ref (rad)/1 -> Terminator/1
  All meas/1 -> Position Controller/4(All_meas), Velocity Controller/4(All_meas), Bus Selector1/1
  Mux2/1 -> Euler des/1
  Mux1/1 -> Accels des/1
  Position Controller/1(Ve des (m/s)) -> Demux2/1
  Demux2/2 -> Velocity Controller/2(Ve_y_ref)
  Demux2/1 -> Velocity Controller/1(Ve_x_ref)
  Demux2/3 -> Velocity Controller/3(Ve_z_ref)
  Velocity Controller/1(Acc_e des (m/s)) -> Yaw rotate/1(Acc_e)
  Bus Selector1/1 -> Selector/1  "<Euler meas (rad)>"
  Selector/1 -> Yaw rotate/2(yaw)
  3D vec norm/1 -> Mux1/2
  Yaw rotate/1(Acc_yaw) -> A_x/1, 3D vec norm/1, A_y/1
  Yaw_ref (rad)/1 -> Mux2/3
  A_y/1 -> Divide/1
  g/1 -> Divide/2, Divide1/1
  A_x/1 -> Divide1/2
  Divide/1 -> Trigonometric Function/1
  Divide1/1 -> Trigonometric Function1/1
  Trigonometric Function1/1 -> Gain/1
  Trigonometric Function/1 -> Mux2/1
  Gain/1 -> Mux2/2

== system Tricopter_Controlled_development/FlightGear visualization/Flat Earth to LLA/ne to lat//long/Latitude Between +//- 90  ==
  mu l : Inport
  Constant1 : Constant  Value=180
  Constant3 : Constant  Value=90
  Constant4 : Constant  Value=180
  Constant5 : Constant  Value=360
  Data Type Conversion : DataTypeConversion
  Demux : Demux  Outputs=2
  Gain : Gain  Gain=180
  Gain1 : Gain  Gain=2
  Gain2 : Gain  Gain=2
  Gain3 : Gain  Gain=360
  Gain4 : Gain  Gain=180
  Logical Operator1 : Logic  AllPortsSameDT=off  OutDataTypeStr=boolean
  Math Function1 : Math  Operator=rem  SaturateOnIntegerOverflow=on
  Math Function2 : Math  Operator=rem  SaturateOnIntegerOverflow=on
  Mux : Mux  Inputs=2
  Product : Product  Inputs=*/  RndMeth=Zero
  Product1 : Product  RndMeth=Zero
  Product2 : Product  Inputs=*/  RndMeth=Zero
  Product3 : Product  RndMeth=Zero
  Rounding Function : Rounding  Operator=fix
  Rounding Function1 : Rounding  Operator=fix
  Rounding Function2 : Rounding  Operator=fix
  Sum1 : Sum  Inputs=|-+
  Sum2 : Sum  Inputs=+--
  Sum3 : Sum  Inputs=++|
  sqrt : Sqrt  AlgorithmType=Newton-Raphson  SaturateOnIntegerOverflow=on
  "mu l " : Outport
  wires:
  Sum3/1 -> Mux/2
  Demux/2 -> Sum3/2
  Demux/1 -> Math Function1/1
  mu l/1 -> Demux/1
  Mux/1 -> "mu l "/1
  Constant1/1 -> Product/2
  Product/1 -> Rounding Function/1, Gain1/1
  Rounding Function/1 -> Gain/1
  Gain/1 -> Sum2/2
  Sum2/1 -> Mux/1
  Constant3/1 -> Math Function2/2
  Math Function2/1 -> Product3/2
  Product3/1 -> Sum2/3
  Rounding Function2/1 -> Gain2/1
  Gain2/1 -> Product3/1, Logical Operator1/1, Logical Operator1/2
  Product1/1 -> sqrt/1
  sqrt/1 -> Rounding Function2/1
  Constant4/1 -> Product2/2
  Product2/1 -> Rounding Function1/1
  Rounding Function1/1 -> Gain3/1
  Gain3/1 -> Sum1/1
  Math Function1/1 -> Sum1/2, Product2/1
  Sum1/1 -> Math Function2/1, Product/1, Sum2/1
  Constant5/1 -> Math Function1/2
  Logical Operator1/1 -> Data Type Conversion/1
  Gain4/1 -> Sum3/1
  Data Type Conversion/1 -> Gain4/1
  Gain1/1 -> Product1/2, Product1/1

== system Tricopter_Controlled_development/FlightGear visualization/Flat Earth to LLA/ne to lat//long/LongLat_offset  ==
  XY : Inport
  mu : Inport  Port=2
  " " : Trigonometry
  "  " : Trigonometry  Operator=cos
  Demux : Demux  Outputs=2
  "Find Radian/Distance " : Subsystem  TreatAsAtomicUnit=on
  Mux : Mux  Inputs=2
  Sum : Sum  Inputs=|+-
  Sum1 : Sum  Inputs=|++
  deg2rad : Gain  Gain=pi/180  SaturateOnIntegerOverflow=on  OutDataTypeStr=Inherit: Same as input  ParamDataTypeStr=Inherit: Same as input
  rad lat : Product  RndMeth=Zero
  "rad long " : Product  RndMeth=Zero
  ref_pos : Constant  Value=0
  x*cos : Product  RndMeth=Zero
  x*sin : Product  RndMeth=Zero
  y*cos : Product  RndMeth=Zero
  y*sin : Product  RndMeth=Zero
  DeltaLL_rad : Outport
  wires:
  mu/1 -> "Find Radian/Distance "/1(mu)
  "Find Radian/Distance "/1(dNorth) -> rad lat/2
  "Find Radian/Distance "/2(dEast) -> "rad long "/1
  rad lat/1 -> Mux/1
  "rad long "/1 -> Mux/2
  Mux/1 -> DeltaLL_rad/1
  deg2rad/1 -> "  "/1, " "/1
  Demux/2 -> y*cos/1, y*sin/1
  Sum1/1 -> "rad long "/2
  y*cos/1 -> Sum1/2
  x*sin/1 -> Sum1/1
  Sum/1 -> rad lat/1
  y*sin/1 -> Sum/2
  " "/1 -> x*sin/2, y*sin/2
  x*cos/1 -> Sum/1
  "  "/1 -> y*cos/2, x*cos/2
  Demux/1 -> x*sin/1, x*cos/1
  XY/1 -> Demux/1
  ref_pos/1 -> deg2rad/1

== system Tricopter_Controlled_development/FlightGear visualization/Flat Earth to LLA/ne to lat//long/Longitude Between +//-180  ==
  mu l : Inport
  Constant : Constant  Value=180
  Constant2 : Constant  Value=360
  Demux1 : Demux  Outputs=2
  Gain : Gain  Gain=360
  Math Function2 : Math  Operator=rem  SaturateOnIntegerOverflow=on
  Mux1 : Mux  Inputs=2
  Product : Product  Inputs=*/  RndMeth=Zero
  Rounding Function : Rounding  Operator=fix
  Sum2 : Sum  Inputs=|-+
  "mu l " : Outport
  wires:
  Mux1/1 -> "mu l "/1
  Demux1/1 -> Mux1/1
  mu l/1 -> Demux1/1
  Constant/1 -> Product/2
  Product/1 -> Rounding Function/1
  Rounding Function/1 -> Gain/1
  Gain/1 -> Sum2/1
  Sum2/1 -> Mux1/2
  Demux1/2 -> Math Function2/1
  Constant2/1 -> Math Function2/2
  Math Function2/1 -> Product/1, Sum2/2

== system Tricopter_Controlled_development/TriCopter FCS development/Inner Controller/P Controller/Attitude Controller ==
  phi_ref : Inport
  theta_ref : Inport  Port=2
  psi_ref : Inport  Port=3
  All_meas : Inport  Port=4
  Bus Creator : BusCreator
  Bus Creator1 : BusCreator
  Bus Creator2 : BusCreator
  Bus Selector : BusSelector  OutputSignals=Meas.Euler meas (rad)
  Mux : Mux  Inputs=3
  Ref Model and P Controller p : Adaptive_FaultTolerantControl/Ref Model and P Controller  tau=1.5  y_i=0  K_f=1  K_b=2
  Ref Model and P Controller q : Adaptive_FaultTolerantControl/Ref Model and P Controller  tau=1.5  y_i=0  K_f=1  K_b=2
  Ref Model and P Controller q1 : Adaptive_FaultTolerantControl/Ref Model and P Controller  tau=5  y_i=0  K_f=0.5  K_b=1
  Selector : Selector  InputPortWidth=3
  Selector1 : Selector  InputPortWidth=3  Indices=2
  Selector2 : Selector  InputPortWidth=3  Indices=3
  Sum : Sum  Inputs=+-|
  Sum1 : Sum  Inputs=+-|
  Sum2 : Sum  Inputs=+-|
  Terminator1 : Terminator
  Terminator2 : Terminator
  Terminator3 : Terminator
  Euler_dot des (rad/s) : Outport
  wires:
  Ref Model and P Controller q1/4 -> Sum2/2
  Sum2/1 -> Bus Creator2/3  "Vz_err"
  Ref Model and P Controller q1/3 -> Bus Creator2/2, Sum2/1  "Vz_sf"
  Ref Model and P Controller q1/2 -> Bus Creator2/1  "Vz_sf_dot"
  Ref Model and P Controller q/5 -> Bus Creator1/4  "K_b_Vy"
  Ref Model and P Controller q/4 -> Sum1/2
  Sum1/1 -> Bus Creator1/3  "Vy_err"
  Ref Model and P Controller q/3 -> Bus Creator1/2, Sum1/1  "Vy_sf"
  Ref Model and P Controller q/2 -> Bus Creator1/1  "Vy_sf_dot"
  Ref Model and P Controller p/5 -> Bus Creator/4  "K_b_Vx"
  Ref Model and P Controller p/4 -> Sum/2
  Selector2/1 -> Ref Model and P Controller q1/2
  Bus Creator2/1 -> Terminator3/1
  Bus Creator1/1 -> Terminator1/1
  Bus Creator/1 -> Terminator2/1
  Sum/1 -> Bus Creator/3  "Vx_err"
  Ref Model and P Controller p/3 -> Bus Creator/2, Sum/1  "Vx_sf"
  Ref Model and P Controller p/2 -> Bus Creator/1  "Vx_sf_dot"
  Ref Model and P Controller q1/1 -> Mux/3
  Ref Model and P Controller q/1 -> Mux/2
  psi_ref/1 -> Ref Model and P Controller q1/1
  Selector1/1 -> Ref Model and P Controller q/2
  theta_ref/1 -> Ref Model and P Controller q/1
  Mux/1 -> Euler_dot des (rad/s)/1
  Ref Model and P Controller p/1 -> Mux/1
  Selector/1 -> Ref Model and P Controller p/2
  phi_ref/1 -> Ref Model and P Controller p/1
  Bus Selector/1 -> Selector2/1, Selector1/1, Selector/1  "<Euler meas (rad)>"
  All_meas/1 -> Bus Selector/1
  Ref Model and P Controller q1/5 -> Bus Creator2/4  "K_b_psi"

== system Tricopter_Controlled_development/TriCopter FCS development/Inner Controller/P Controller/Body Rates Controller ==
  p_ref : Inport
  q_ref : Inport  Port=2
  r_ref : Inport  Port=3
  All_meas : Inport  Port=4
  Bus Creator : BusCreator
  Bus Creator1 : BusCreator
  Bus Creator2 : BusCreator
  Bus Selector : BusSelector  OutputSignals=Meas.omega_b meas (rad/s)
  Mux : Mux  Inputs=3
  Ref Model and P Controller p : Adaptive_FaultTolerantControl/Ref Model and P Controller  tau=0.7  y_i=0  K_f=1  K_b=5
  Ref Model and P Controller q : Adaptive_FaultTolerantControl/Ref Model and P Controller  tau=0.7  y_i=0  K_f=1  K_b=5
  Ref Model and P Controller r : Adaptive_FaultTolerantControl/Ref Model and P Controller  tau=1.5  y_i=0  K_f=1  K_b=3
  Saturation : Saturate  UpperLimit=0.1  LowerLimit=-0.1
  Selector : Selector  InputPortWidth=3
  Selector1 : Selector  InputPortWidth=3  Indices=2
  Selector2 : Selector  InputPortWidth=3  Indices=3
  Sum : Sum  Inputs=+-|
  Sum1 : Sum  Inputs=+-|
  Sum2 : Sum  Inputs=+-|
  Terminator1 : Terminator
  Terminator2 : Terminator
  Terminator3 : Terminator
  Angular acc des (rad/s^2) : Outport
  wires:
  Ref Model and P Controller r/5 -> Bus Creator2/4  "K_b_r"
  Ref Model and P Controller r/4 -> Sum2/2
  Sum2/1 -> Bus Creator2/3  "r_err"
  Ref Model and P Controller r/3 -> Bus Creator2/2, Sum2/1  "r_sf"
  Ref Model and P Controller r/2 -> Bus Creator2/1  "r_sf_dot"
  Ref Model and P Controller q/5 -> Bus Creator1/4  "K_b_q"
  Ref Model and P Controller q/4 -> Sum1/2
  Sum1/1 -> Bus Creator1/3  "q_err"
  Ref Model and P Controller q/3 -> Bus Creator1/2, Sum1/1  "q_sf"
  Ref Model and P Controller q/2 -> Bus Creator1/1  "q_sf_dot"
  Ref Model and P Controller p/5 -> Bus Creator/4  "K_b_p"
  Ref Model and P Controller p/4 -> Sum/2
  Selector2/1 -> Ref Model and P Controller r/2
  Bus Creator2/1 -> Terminator3/1
  Bus Creator1/1 -> Terminator1/1
  Bus Creator/1 -> Terminator2/1
  Sum/1 -> Bus Creator/3  "p_err"
  Ref Model and P Controller p/3 -> Bus Creator/2, Sum/1  "p_sf"
  Ref Model and P Controller p/2 -> Bus Creator/1  "p_sf_dot"
  Ref Model and P Controller r/1 -> Saturation/1
  r_ref/1 -> Ref Model and P Controller r/1
  Selector1/1 -> Ref Model and P Controller q/2
  q_ref/1 -> Ref Model and P Controller q/1
  Mux/1 -> Angular acc des (rad/s^2)/1
  Selector/1 -> Ref Model and P Controller p/2
  p_ref/1 -> Ref Model and P Controller p/1
  Bus Selector/1 -> Selector2/1, Selector1/1, Selector/1  "<omega_b meas (rad/s)>"
  All_meas/1 -> Bus Selector/1
  Saturation/1 -> Mux/3
  Ref Model and P Controller q/1 -> Mux/2
  Ref Model and P Controller p/1 -> Mux/1

== system Tricopter_Controlled_development/TriCopter FCS development/Inner Controller/PI Controller/Attitude Controller ==
  phi_ref : Inport
  theta_ref : Inport  Port=2
  psi_ref : Inport  Port=3
  All_meas : Inport  Port=4
  Bus Creator : BusCreator
  Bus Creator1 : BusCreator
  Bus Creator2 : BusCreator
  Bus Selector : BusSelector  OutputSignals=Meas.Euler meas (rad)
  Mux : Mux  Inputs=3
  Ref Model and PI Controller : Adaptive_FaultTolerantControl/Ref Model and PI Controller  delta=0  tau=5  y_i=0  K_f=0  K_a=1  Con_way=pro  omega_n=4  xi=0.5  Z1=-30  K_b=2  f_i=0.2  f_c=1
  Ref Model and PI Controller1 : Adaptive_FaultTolerantControl/Ref Model and PI Controller  delta=0  tau=5  y_i=0  K_f=0  K_a=1  Con_way=pro  omega_n=4  xi=0.5  Z1=-30  K_b=3  f_i=0.2  f_c=1
  Ref Model and PI Controller2 : Adaptive_FaultTolerantControl/Ref Model and PI Controller  delta=0  tau=1  y_i=0  K_f=0  K_a=1  Con_way=pro  omega_n=4  xi=0.5  Z1=-30  K_b=3  f_i=0.2  f_c=1
  Selector : Selector  InputPortWidth=3
  Selector1 : Selector  InputPortWidth=3  Indices=2
  Selector2 : Selector  InputPortWidth=3  Indices=3
  Sum : Sum  Inputs=+-|
  Sum1 : Sum  Inputs=+-|
  Sum2 : Sum  Inputs=+-|
  Terminator1 : Terminator
  Terminator2 : Terminator
  Terminator3 : Terminator
  Euler_dot des (rad/s) : Outport
  wires:
  All_meas/1 -> Bus Selector/1
  Bus Selector/1 -> Selector1/1, Selector/1, Selector2/1  "<Euler meas (rad)>"
  phi_ref/1 -> Ref Model and PI Controller2/1
  Selector/1 -> Ref Model and PI Controller2/2
  Ref Model and PI Controller2/1 -> Mux/1
  Mux/1 -> Euler_dot des (rad/s)/1
  theta_ref/1 -> Ref Model and PI Controller1/1
  Selector1/1 -> Ref Model and PI Controller1/2
  psi_ref/1 -> Ref Model and PI Controller/1
  Ref Model and PI Controller1/1 -> Mux/2
  Ref Model and PI Controller/1 -> Mux/3
  Ref Model and PI Controller2/2 -> Bus Creator/1  "Vx_sf_dot"
  Ref Model and PI Controller2/3 -> Bus Creator/2, Sum/1  "Vx_sf"
  Sum/1 -> Bus Creator/3  "Vx_err"
  Bus Creator/1 -> Terminator2/1
  Bus Creator1/1 -> Terminator1/1
  Bus Creator2/1 -> Terminator3/1
  Selector2/1 -> Ref Model and PI Controller/2
  Ref Model and PI Controller2/4 -> Sum/2
  Ref Model and PI Controller1/2 -> Bus Creator1/1  "Vy_sf_dot"
  Ref Model and PI Controller1/3 -> Bus Creator1/2, Sum1/1  "Vy_sf"
  Sum1/1 -> Bus Creator1/3  "Vy_err"
  Ref Model and PI Controller1/4 -> Sum1/2
  Ref Model and PI Controller/2 -> Bus Creator2/1  "Vz_sf_dot"
  Ref Model and PI Controller/3 -> Sum2/1, Bus Creator2/2  "Vz_sf"
  Sum2/1 -> Bus Creator2/3  "Vz_err"
  Ref Model and PI Controller/4 -> Sum2/2

== system Tricopter_Controlled_development/TriCopter FCS development/Inner Controller/PI Controller/Body Rates Controller ==
  p_ref : Inport
  q_ref : Inport  Port=2
  r_ref : Inport  Port=3
  All_meas : Inport  Port=4
  Bus Creator : BusCreator
  Bus Creator1 : BusCreator
  Bus Creator2 : BusCreator
  Bus Selector : BusSelector  OutputSignals=Meas.omega_b meas (rad/s)
  Mux : Mux  Inputs=3
  Ref Model and P Controller p : Adaptive_FaultTolerantControl/Ref Model and P Controller  tau=0.7  y_i=0  K_f=0.7  K_b=3
  Ref Model and P Controller q : Adaptive_FaultTolerantControl/Ref Model and P Controller  tau=0.7  y_i=0  K_f=0.7  K_b=3
  Ref Model and P Controller r : Adaptive_FaultTolerantControl/Ref Model and P Controller  tau=2  y_i=0  K_f=0.7  K_b=1.2
  Selector : Selector  InputPortWidth=3
  Selector1 : Selector  InputPortWidth=3  Indices=2
  Selector2 : Selector  InputPortWidth=3  Indices=3
  Sum : Sum  Inputs=+-|
  Sum1 : Sum  Inputs=+-|
  Sum2 : Sum  Inputs=+-|
  Terminator1 : Terminator
  Terminator2 : Terminator
  Terminator3 : Terminator
  Angular acc des (rad/s^2) : Outport
  wires:
  Ref Model and P Controller p/1 -> Mux/1
  Ref Model and P Controller q/1 -> Mux/2
  Ref Model and P Controller r/1 -> Mux/3
  All_meas/1 -> Bus Selector/1
  Bus Selector/1 -> Selector/1, Selector1/1, Selector2/1  "<omega_b meas (rad/s)>"
  p_ref/1 -> Ref Model and P Controller p/1
  Selector/1 -> Ref Model and P Controller p/2
  Mux/1 -> Angular acc des (rad/s^2)/1
  q_ref/1 -> Ref Model and P Controller q/1
  Selector1/1 -> Ref Model and P Controller q/2
  r_ref/1 -> Ref Model and P Controller r/1
  Ref Model and P Controller p/2 -> Bus Creator/1  "p_sf_dot"
  Ref Model and P Controller p/3 -> Sum/1, Bus Creator/2  "p_sf"
  Sum/1 -> Bus Creator/3  "p_err"
  Bus Creator/1 -> Terminator2/1
  Bus Creator1/1 -> Terminator1/1
  Bus Creator2/1 -> Terminator3/1
  Selector2/1 -> Ref Model and P Controller r/2
  Ref Model and P Controller p/4 -> Sum/2
  Ref Model and P Controller p/5 -> Bus Creator/4  "K_b_p"
  Ref Model and P Controller q/2 -> Bus Creator1/1  "q_sf_dot"
  Ref Model and P Controller q/3 -> Sum1/1, Bus Creator1/2  "q_sf"
  Sum1/1 -> Bus Creator1/3  "q_err"
  Ref Model and P Controller q/4 -> Sum1/2
  Ref Model and P Controller q/5 -> Bus Creator1/4  "K_b_q"
  Ref Model and P Controller r/2 -> Bus Creator2/1  "r_sf_dot"
  Ref Model and P Controller r/3 -> Sum2/1, Bus Creator2/2  "r_sf"
  Sum2/1 -> Bus Creator2/3  "r_err"
  Ref Model and P Controller r/4 -> Sum2/2
  Ref Model and P Controller r/5 -> Bus Creator2/4  "K_b_r"

== system Tricopter_Controlled_development/TriCopter FCS development/Inner Controller/PI Controller/Limits in Ang accel ==
  note: Here it is assumed that at all time every prop is generating m*g/3 newtons of force . It is conservative?
  Ang Ace des : Inport
  Euler meas : Inport  Port=2
  Limis eval : MATLAB Function  TreatAsAtomicUnit=on
  Saturation Dynamic : simulink/Discontinuities/Saturation Dynamic  OutMin=[]  OutMax=[]  OutDataTypeStr=Inherit: Same as second input  OutDataType=fixdt(1, 16)  OutScaling=2^-10  DoSatur=off
  ang Ace des : Outport
  wires:
  Limis eval/1(Limit_up) -> Saturation Dynamic/1
  Limis eval/2(Limit_down) -> Saturation Dynamic/3
  Euler meas/1 -> Limis eval/2(euler_ang)
  Ang Ace des/1 -> Saturation Dynamic/2, Limis eval/1(Ang_Accel)
  Saturation Dynamic/1 -> ang Ace des/1

== system Tricopter_Controlled_development/TriCopter FCS development/Inner Controller/PI Controller/keep -pi//pi1 ==
  in (rad) : Inport
  Constant : Constant  Value=180
  Constant2 : Constant  Value=360
  Gain : Gain  Gain=360
  Math Function2 : Math  Operator=rem  SaturateOnIntegerOverflow=on
  Product : Product  Inputs=*/  RndMeth=Zero
  Rounding Function : Rounding  Operator=fix
  Sum2 : Sum  Inputs=|-+
  deg2rad1 : Gain  Gain=pi/180  SaturateOnIntegerOverflow=on  OutDataTypeStr=Inherit: Same as input  ParamDataTypeStr=Inherit: Same as input
  rad2deg : Gain  Gain=180/pi  SaturateOnIntegerOverflow=on  OutDataTypeStr=Inherit: Same as input  ParamDataTypeStr=Inherit: Same as input
  out (rad) : Outport
  wires:
  in (rad)/1 -> rad2deg/1
  Constant/1 -> Product/2
  Product/1 -> Rounding Function/1
  Rounding Function/1 -> Gain/1
  Gain/1 -> Sum2/1
  rad2deg/1 -> Math Function2/1
  Constant2/1 -> Math Function2/2
  Math Function2/1 -> Product/1, Sum2/2
  Sum2/1 -> deg2rad1/1
  deg2rad1/1 -> out (rad)/1
